simulink model "sensor_step_response"  (R2022a)
settings: Solver=VariableStepAuto  StartTime=0.0  StopTime=20  RelTol=1e-3
values from neighbouring files (symbols this model uses):
  k = 1.2    [run_frequency_sweep.m]
  r = 0.2    [run_frequency_sweep.m]
  x0 = 0    [measure_frequency_point.m]
  y0 = 0    [measure_frequency_point.m]
settings Model: Creator=HJL  LastModifiedBy=HJL

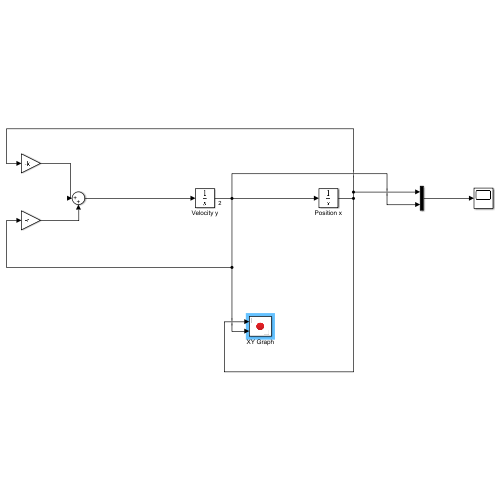
[thumbnail: Simulink's stored preview of the top-level diagram]
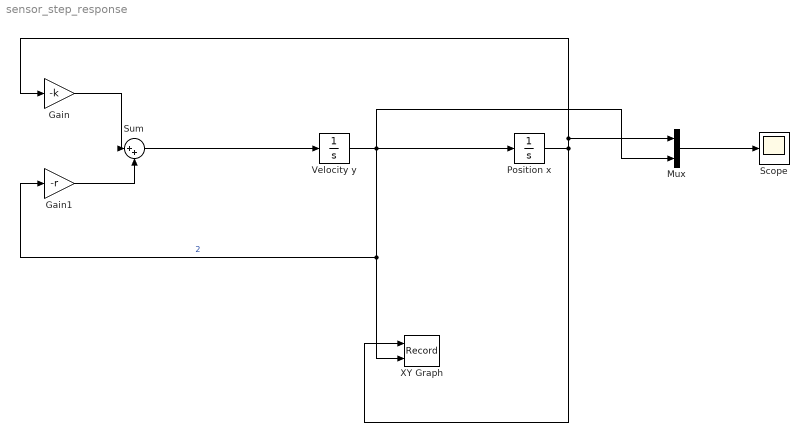
== system sensor_step_response ==
  Gain : Gain  Gain=-k
  Gain1 : Gain  Gain=-r
  Mux : Mux  Inputs=2
  Position x : Integrator  InitialCondition=x0
  Scope : Scope
  Sum : Sum  Inputs=|++
  Velocity y : Integrator  InitialCondition=y0
  XY Graph : Record  FileSettingsInternal="{\"entries\":[{\"content\":{\"excelSettings\":{\"content\":{},\"type\":\"Streamout.ExcelSettings\"}},\"type\":\"Streamout.FileSettingStorage\",\"uuid\":\"4bbe66f4-e25d-4b2c-b27d-b603bd20275e\"}],\"packageUris\":[\"http://schema.mathworks.com/mf0/streamout_blocks/R2020a\"],\"version\":\"1.0\"}"  Layout=[1 1]  SignalsInternal="{\"entries\":[{\"content\":{\"signals\":[{\"content\":{\"blockPath\":[\"harmonic_oscillator_demo/XY Graph\"],\"channel\":[],\"dimensions\":[1],\"domain\":\"harmonic_oscillator_demo/XY Graph\",\"lineColor\":\"#a2142f\",\"plots\":[1],\"port\":1,\"sid\":[\"\"],\"signalID\":123,\"signalName\":\"Position x\"},\"type\":\"RecordBlkView.Signal\",\"uuid\":\"dee94f5c-36c0-4e3f-b58d-db5ec21e1ea3\"},{\"content\":{\"blockPath\":[\"harmonic_oscillator_demo/XY Graph\"],\"channel\":[],\"dimensions\":[1],\"domain\":\"harmonic_oscillator_demo/XY Graph\",\"lineColor\":\"#139fff\",\"plots\":[1],\"port\":2,\"sid\":[\"\"],\"signalID\":127,\"signalName\":\"2\"},\"type\":\"RecordBlkView.Signal\",\"uuid\":\"9c9d3442-7a8d-4678-b419-6159aa415496\"}]},\"type\":\"RecordBlkView.InputSignals\",\"uuid\":\"1a1318ca-0213-48d4-b097-b257e54db5d4\"}],\"packageUris\":[\"http://schema.mathworks.com/mf0/streamout_blocks/R2020a\"],\"version\":\"1.0\"}"  VisualizationBindings="{\"xyplotplugin\":{\"info\":[{\"series\":[{\"bindingParametersList\":[{\"parameter\":\"X-Axis\",\"signalID\":123,\"signalName\":\"Position x\"},{\"parameter\":\"Y-Axis\",\"signalID\":127,\"signalName\":\"2\"}],\"seriesID\":21724}],\"subplotID\":1}]}}"  CompatibilityTag=XY
  wires:
  Gain1/1 -> Sum/2
  Gain/1 -> Sum/1
  Sum/1 -> Velocity y/1
  Position x/1 -> Mux/1, Gain/1, XY Graph/1
  Velocity y/1 -> XY Graph/2, Gain1/1, Mux/2, Position x/1  "2"
  Mux/1 -> Scope/1
